simulink model "SPM_Pack"  (R2024b)
settings: Solver=VariableStepAuto  StartTime=0.0  StopTime=10.0  RelTol=1e-3
libraries: fl_lib x74, nesl_utility x33, batt_lib x8, BatteryEstimators x8, ee_lib x8
(part 1 of 2)
settings Model: Creator=annaf  LastModifiedBy=annaf

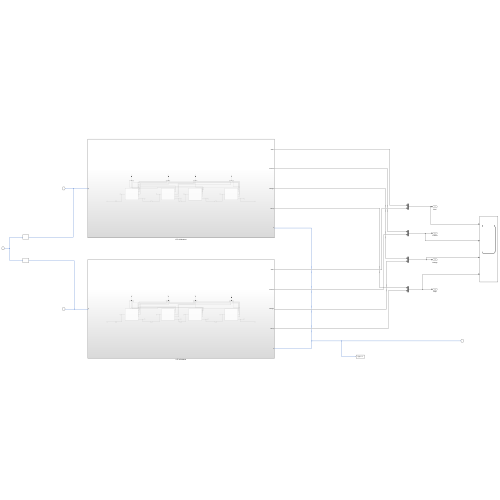
[thumbnail: Simulink's stored preview of the top-level diagram]
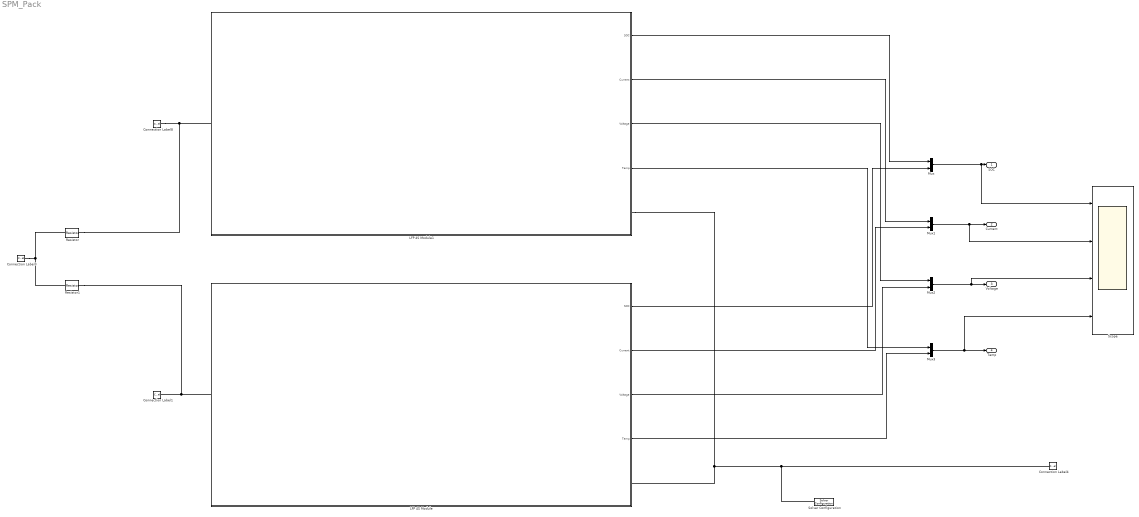
== system SPM_Pack ==
  Connection Label1 : ConnectionLabel  Label=p
  Connection Label3 : ConnectionLabel  Label=p
  Connection Label4 : ConnectionLabel  Label=n
  Connection Label8 : ConnectionLabel  Label=p
  LFP 4S Module : Subsystem
  LFP 4S Module1 : Subsystem
  Mux{,1..3} (4 alike) : Mux  Inputs=2
  Resistor : fl_lib/Electrical/Electrical Elements/Resistor  R=0.001 Ohm  i_specify=off  i_priority=None  i=0 A  i_nominal_specify=off  i_nominal_value=1  i_nominal_unit=A  v_specify=off  v_priority=None  v=0 V  v_nominal_specify=off  v_nominal_value=1  v_nominal_unit=V
  Resistor1 : fl_lib/Electrical/Electrical Elements/Resistor  R=0.001 Ohm  i_specify=off  i_priority=None  i=0 A  i_nominal_specify=off  i_nominal_value=1  i_nominal_unit=A  v_specify=off  v_priority=None  v=0 V  v_nominal_specify=off  v_nominal_value=1  v_nominal_unit=V
  Scope : Scope  NumInputPorts=4
  Solver Configuration : nesl_utility/Solver Configuration  PhysicalDomain=network_engine_domain  SubClassName=solver  LeftPortType=input  RightPortType=generic  Tones=[]  Harmonics=[]  SimulateNoise=off  Profile=off  UseLocalSampling=off  EnableSwitchedLinearOptims=on  FrequencyDomain=off  UseCCode=off  RelTol=0.001  AbsTol=0.001  MinStep=1e-09  ToWorkspace=off  RevertToSquareIcSolve=off  NumHomotopyIterations=100  PhasorMode=off  PhasorModeNumHarmonics=1  ConsistencySolver=NEWTON_XTOL_AFTER_FTOL  IndexReductionMethod=DerivativeReplacement  DoDC=off  ResidualTolerance=1e-09  ConsistencyTolSource=GLOBAL  ConsistencyAbsTol=0.001  ConsistencyRelTol=0.001  ConsistencyTolFactor=0.001  UseLocalSolver=on  LocalSolverChoice=NE_BACKWARD_EULER_ADVANCER  ResolveIndetEquations=off  FunctionEvalNumThread=1  LocalSolverSampleTime=0.1  DoFixedCost=off  MaxNonlinIter=3  MaxModeIter=2  ComputeImpulses=off  ImpulseIterations=2  LinearAlgebra=auto  LinearAlgebraNumThread=0  EquationFormulation=NE_TIME_EF  DelaysMemoryBudget=1024  AutomaticFiltering=on  FilteringTimeConstant=0.001  PartitionStorageMethod=AS_NEEDED  PartitionMemoryBudget=1024  PartitionMethod=ROBUST  MultibodyUseLocalSolver=off  MultibodyLocalSolverChoice=ODE1  MultibodyLocalSolverSampleTime=0.001
  SOC : Outport
  Current : Outport  Port=2
  Voltage : Outport  Port=3
  Temp : Outport  Port=4
  wires:
  Mux2/1 -> Scope/3, Voltage/1
  Mux1/1 -> Scope/2, Current/1
  Mux/1 -> Scope/1, SOC/1
  Mux3/1 -> Scope/4, Temp/1
  LFP 4S Module1/1(SOC) -> Mux/1
  LFP 4S Module/1(SOC) -> Mux/2
  LFP 4S Module1/2(Current) -> Mux1/1
  LFP 4S Module1/3(Voltage) -> Mux2/1
  LFP 4S Module1/4(Temp) -> Mux3/1
  LFP 4S Module/2(Current) -> Mux1/2
  LFP 4S Module/3(Voltage) -> Mux2/2
  LFP 4S Module/4(Temp) -> Mux3/2
  connections:
  Connection Label8/LConn1 -- Resistor/RConn1 -- LFP 4S Module1/LConn1
  LFP 4S Module1/RConn1 -- Solver Configuration/RConn1 -- Connection Label4/LConn1 -- LFP 4S Module/RConn1
  LFP 4S Module/LConn1 -- Resistor1/RConn1 -- Connection Label1/LConn1
  Resistor1/LConn1 -- Connection Label3/LConn1 -- Resistor/LConn1

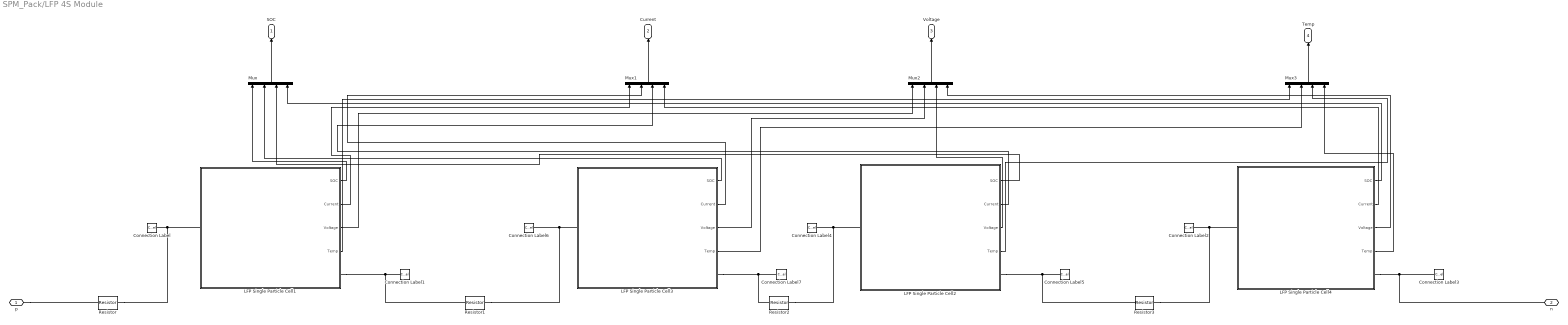
== system SPM_Pack/LFP 4S Module ==
  Connection Label{,2,4,6} (4 alike) : ConnectionLabel  Label=p
  Connection Label{1,3,5,7} (4 alike) : ConnectionLabel  Label=n
  LFP Single Particle Cell1 : Subsystem
  LFP Single Particle Cell2 : Subsystem
  LFP Single Particle Cell3 : Subsystem
  LFP Single Particle Cell4 : Subsystem
  Mux{,1..3} (4 alike) : Mux
  Resistor : ee_lib/Passive/Resistor  R=0.002 Ohm  enable_R_tol=ee.enum.toleranceApplication.none  R_tol=5  tol_distribution=ee.enum.toleranceDistribution.uniform  nSigma=4  enable_operating_limits=ee.enum.enable.no  operating_limit_action=ee.enum.passive.reportOpLim.warn  power_rating=1 W  max_working_voltage=100 V  noise_mode=ee.enum.sources.noise.Disabled  Tdevice=25 degC  sample_time=1e-3 s  repeatability=ee.enum.ic.repeatability.notRepeatable  user_seed=0  auto_seed=4144164703  fault_action=simscape.enum.assert.action.none  t_fault=1 s  power_derating_T1=70 degC  power_derating_T2=155 degC  operating_temperature_range_vec=[-50, 150] degC  alpha=3.93e-3 1/K  Tmeas=25 degC  thermal_mass=100 J/K  temperature_specify=off  temperature_priority=High  temperature=298.15 K  temperature_nominal_specify=off  temperature_nominal_value=1  temperature_nominal_unit=K
  Resistor1 : ee_lib/Passive/Resistor  R=0.002 Ohm  enable_R_tol=ee.enum.toleranceApplication.none  R_tol=5  tol_distribution=ee.enum.toleranceDistribution.uniform  nSigma=4  enable_operating_limits=ee.enum.enable.no  operating_limit_action=ee.enum.passive.reportOpLim.warn  power_rating=1 W  max_working_voltage=100 V  noise_mode=ee.enum.sources.noise.Disabled  Tdevice=25 degC  sample_time=1e-3 s  repeatability=ee.enum.ic.repeatability.notRepeatable  user_seed=0  auto_seed=676943032  fault_action=simscape.enum.assert.action.none  t_fault=1 s  power_derating_T1=70 degC  power_derating_T2=155 degC  operating_temperature_range_vec=[-50, 150] degC  alpha=3.93e-3 1/K  Tmeas=25 degC  thermal_mass=100 J/K  temperature_specify=off  temperature_priority=High  temperature=298.15 K  temperature_nominal_specify=off  temperature_nominal_value=1  temperature_nominal_unit=K
  Resistor2 : ee_lib/Passive/Resistor  R=0.002 Ohm  enable_R_tol=ee.enum.toleranceApplication.none  R_tol=5  tol_distribution=ee.enum.toleranceDistribution.uniform  nSigma=4  enable_operating_limits=ee.enum.enable.no  operating_limit_action=ee.enum.passive.reportOpLim.warn  power_rating=1 W  max_working_voltage=100 V  noise_mode=ee.enum.sources.noise.Disabled  Tdevice=25 degC  sample_time=1e-3 s  repeatability=ee.enum.ic.repeatability.notRepeatable  user_seed=0  auto_seed=4168664255  fault_action=simscape.enum.assert.action.none  t_fault=1 s  power_derating_T1=70 degC  power_derating_T2=155 degC  operating_temperature_range_vec=[-50, 150] degC  alpha=3.93e-3 1/K  Tmeas=25 degC  thermal_mass=100 J/K  temperature_specify=off  temperature_priority=High  temperature=298.15 K  temperature_nominal_specify=off  temperature_nominal_value=1  temperature_nominal_unit=K
  Resistor3 : ee_lib/Passive/Resistor  R=0.002 Ohm  enable_R_tol=ee.enum.toleranceApplication.none  R_tol=5  tol_distribution=ee.enum.toleranceDistribution.uniform  nSigma=4  enable_operating_limits=ee.enum.enable.no  operating_limit_action=ee.enum.passive.reportOpLim.warn  power_rating=1 W  max_working_voltage=100 V  noise_mode=ee.enum.sources.noise.Disabled  Tdevice=25 degC  sample_time=1e-3 s  repeatability=ee.enum.ic.repeatability.notRepeatable  user_seed=0  auto_seed=4111000739  fault_action=simscape.enum.assert.action.none  t_fault=1 s  power_derating_T1=70 degC  power_derating_T2=155 degC  operating_temperature_range_vec=[-50, 150] degC  alpha=3.93e-3 1/K  Tmeas=25 degC  thermal_mass=100 J/K  temperature_specify=off  temperature_priority=High  temperature=298.15 K  temperature_nominal_specify=off  temperature_nominal_value=1  temperature_nominal_unit=K
  p : PMIOPort  Side=Left
  n : PMIOPort  Port=2  Side=Right
  SOC : Outport
  Current : Outport  Port=2
  Voltage : Outport  Port=3
  Temp : Outport  Port=4
  wires:
  LFP Single Particle Cell1/1(SOC) -> Mux/1
  LFP Single Particle Cell4/4(Temp) -> Mux3/4
  LFP Single Particle Cell2/3(Voltage) -> Mux2/3
  LFP Single Particle Cell3/2(Current) -> Mux1/2
  LFP Single Particle Cell1/2(Current) -> Mux1/1
  LFP Single Particle Cell1/3(Voltage) -> Mux2/1
  LFP Single Particle Cell4/3(Voltage) -> Mux2/4
  LFP Single Particle Cell2/4(Temp) -> Mux3/3
  Mux3/1 -> Temp/1
  LFP Single Particle Cell4/1(SOC) -> Mux/4
  LFP Single Particle Cell2/1(SOC) -> Mux/3
  LFP Single Particle Cell3/3(Voltage) -> Mux2/2
  Mux/1 -> SOC/1
  LFP Single Particle Cell2/2(Current) -> Mux1/3
  LFP Single Particle Cell4/2(Current) -> Mux1/4
  LFP Single Particle Cell3/4(Temp) -> Mux3/2
  Mux2/1 -> Voltage/1
  Mux1/1 -> Current/1
  LFP Single Particle Cell3/1(SOC) -> Mux/2
  LFP Single Particle Cell1/4(Temp) -> Mux3/1
  connections:
  LFP Single Particle Cell4/RConn1 -- Connection Label3/LConn1 -- n/RConn1
  LFP Single Particle Cell3/RConn1 -- Connection Label7/LConn1 -- Resistor2/LConn1
  LFP Single Particle Cell2/LConn1 -- Connection Label4/LConn1 -- Resistor2/RConn1
  LFP Single Particle Cell1/LConn1 -- Connection Label/LConn1 -- Resistor/RConn1
  LFP Single Particle Cell4/LConn1 -- Connection Label2/LConn1 -- Resistor3/RConn1
  LFP Single Particle Cell1/RConn1 -- Connection Label1/LConn1 -- Resistor1/LConn1
  LFP Single Particle Cell3/LConn1 -- Connection Label6/LConn1 -- Resistor1/RConn1
  LFP Single Particle Cell2/RConn1 -- Connection Label5/LConn1 -- Resistor3/LConn1
  p/RConn1 -- Resistor/LConn1

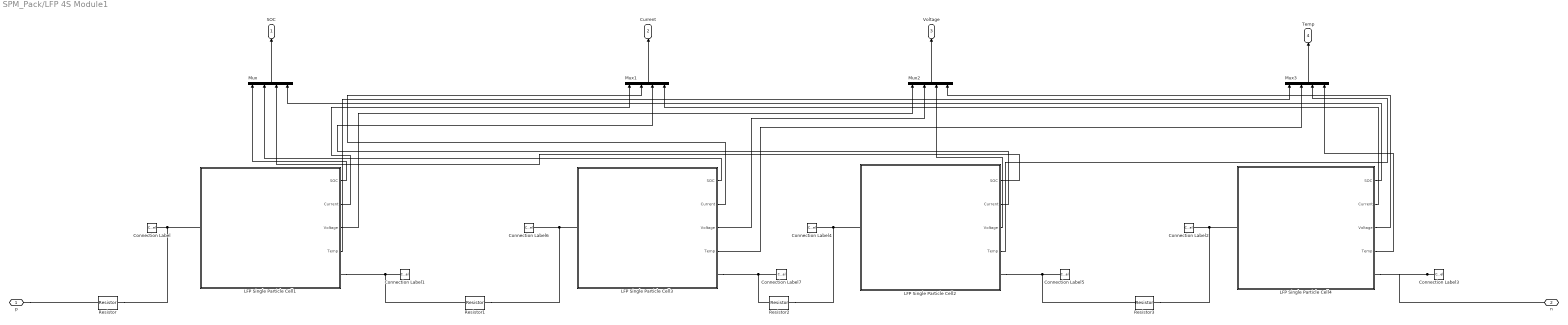
== system SPM_Pack/LFP 4S Module1 ==
  Connection Label{,2,4,6} (4 alike) : ConnectionLabel  Label=p
  Connection Label{1,3,5,7} (4 alike) : ConnectionLabel  Label=n
  LFP Single Particle Cell1 : Subsystem
  LFP Single Particle Cell2 : Subsystem
  LFP Single Particle Cell3 : Subsystem
  LFP Single Particle Cell4 : Subsystem
  Mux{,1..3} (4 alike) : Mux
  Resistor : ee_lib/Passive/Resistor  R=0.002 Ohm  enable_R_tol=ee.enum.toleranceApplication.none  R_tol=5  tol_distribution=ee.enum.toleranceDistribution.uniform  nSigma=4  enable_operating_limits=ee.enum.enable.no  operating_limit_action=ee.enum.passive.reportOpLim.warn  power_rating=1 W  max_working_voltage=100 V  noise_mode=ee.enum.sources.noise.Disabled  Tdevice=25 degC  sample_time=1e-3 s  repeatability=ee.enum.ic.repeatability.notRepeatable  user_seed=0  auto_seed=418932850  fault_action=simscape.enum.assert.action.none  t_fault=1 s  power_derating_T1=70 degC  power_derating_T2=155 degC  operating_temperature_range_vec=[-50, 150] degC  alpha=3.93e-3 1/K  Tmeas=25 degC  thermal_mass=100 J/K  temperature_specify=off  temperature_priority=High  temperature=298.15 K  temperature_nominal_specify=off  temperature_nominal_value=1  temperature_nominal_unit=K
  Resistor1 : ee_lib/Passive/Resistor  R=0.002 Ohm  enable_R_tol=ee.enum.toleranceApplication.none  R_tol=5  tol_distribution=ee.enum.toleranceDistribution.uniform  nSigma=4  enable_operating_limits=ee.enum.enable.no  operating_limit_action=ee.enum.passive.reportOpLim.warn  power_rating=1 W  max_working_voltage=100 V  noise_mode=ee.enum.sources.noise.Disabled  Tdevice=25 degC  sample_time=1e-3 s  repeatability=ee.enum.ic.repeatability.notRepeatable  user_seed=0  auto_seed=1196140742  fault_action=simscape.enum.assert.action.none  t_fault=1 s  power_derating_T1=70 degC  power_derating_T2=155 degC  operating_temperature_range_vec=[-50, 150] degC  alpha=3.93e-3 1/K  Tmeas=25 degC  thermal_mass=100 J/K  temperature_specify=off  temperature_priority=High  temperature=298.15 K  temperature_nominal_specify=off  temperature_nominal_value=1  temperature_nominal_unit=K
  Resistor2 : ee_lib/Passive/Resistor  R=0.002 Ohm  enable_R_tol=ee.enum.toleranceApplication.none  R_tol=5  tol_distribution=ee.enum.toleranceDistribution.uniform  nSigma=4  enable_operating_limits=ee.enum.enable.no  operating_limit_action=ee.enum.passive.reportOpLim.warn  power_rating=1 W  max_working_voltage=100 V  noise_mode=ee.enum.sources.noise.Disabled  Tdevice=25 degC  sample_time=1e-3 s  repeatability=ee.enum.ic.repeatability.notRepeatable  user_seed=0  auto_seed=2348838240  fault_action=simscape.enum.assert.action.none  t_fault=1 s  power_derating_T1=70 degC  power_derating_T2=155 degC  operating_temperature_range_vec=[-50, 150] degC  alpha=3.93e-3 1/K  Tmeas=25 degC  thermal_mass=100 J/K  temperature_specify=off  temperature_priority=High  temperature=298.15 K  temperature_nominal_specify=off  temperature_nominal_value=1  temperature_nominal_unit=K
  Resistor3 : ee_lib/Passive/Resistor  R=0.002 Ohm  enable_R_tol=ee.enum.toleranceApplication.none  R_tol=5  tol_distribution=ee.enum.toleranceDistribution.uniform  nSigma=4  enable_operating_limits=ee.enum.enable.no  operating_limit_action=ee.enum.passive.reportOpLim.warn  power_rating=1 W  max_working_voltage=100 V  noise_mode=ee.enum.sources.noise.Disabled  Tdevice=25 degC  sample_time=1e-3 s  repeatability=ee.enum.ic.repeatability.notRepeatable  user_seed=0  auto_seed=4112460543  fault_action=simscape.enum.assert.action.none  t_fault=1 s  power_derating_T1=70 degC  power_derating_T2=155 degC  operating_temperature_range_vec=[-50, 150] degC  alpha=3.93e-3 1/K  Tmeas=25 degC  thermal_mass=100 J/K  temperature_specify=off  temperature_priority=High  temperature=298.15 K  temperature_nominal_specify=off  temperature_nominal_value=1  temperature_nominal_unit=K
  p : PMIOPort  Side=Left
  n : PMIOPort  Port=2  Side=Right
  SOC : Outport
  Current : Outport  Port=2
  Voltage : Outport  Port=3
  Temp : Outport  Port=4
  wires:
  LFP Single Particle Cell1/1(SOC) -> Mux/1
  LFP Single Particle Cell4/4(Temp) -> Mux3/4
  LFP Single Particle Cell2/3(Voltage) -> Mux2/3
  LFP Single Particle Cell3/2(Current) -> Mux1/2
  LFP Single Particle Cell1/2(Current) -> Mux1/1
  LFP Single Particle Cell1/3(Voltage) -> Mux2/1
  LFP Single Particle Cell4/3(Voltage) -> Mux2/4
  LFP Single Particle Cell2/4(Temp) -> Mux3/3
  Mux3/1 -> Temp/1
  LFP Single Particle Cell4/1(SOC) -> Mux/4
  LFP Single Particle Cell2/1(SOC) -> Mux/3
  LFP Single Particle Cell3/3(Voltage) -> Mux2/2
  Mux/1 -> SOC/1
  LFP Single Particle Cell2/2(Current) -> Mux1/3
  LFP Single Particle Cell4/2(Current) -> Mux1/4
  LFP Single Particle Cell3/4(Temp) -> Mux3/2
  Mux2/1 -> Voltage/1
  Mux1/1 -> Current/1
  LFP Single Particle Cell3/1(SOC) -> Mux/2
  LFP Single Particle Cell1/4(Temp) -> Mux3/1
  connections:
  Connection Label3/LConn1 -- n/RConn1 -- LFP Single Particle Cell4/RConn1
  LFP Single Particle Cell3/RConn1 -- Resistor2/LConn1 -- Connection Label7/LConn1
  LFP Single Particle Cell2/LConn1 -- Resistor2/RConn1 -- Connection Label4/LConn1
  LFP Single Particle Cell1/LConn1 -- Resistor/RConn1 -- Connection Label/LConn1
  LFP Single Particle Cell4/LConn1 -- Resistor3/RConn1 -- Connection Label2/LConn1
  LFP Single Particle Cell1/RConn1 -- Resistor1/LConn1 -- Connection Label1/LConn1
  LFP Single Particle Cell3/LConn1 -- Resistor1/RConn1 -- Connection Label6/LConn1
  LFP Single Particle Cell2/RConn1 -- Resistor3/LConn1 -- Connection Label5/LConn1
  p/RConn1 -- Resistor/LConn1

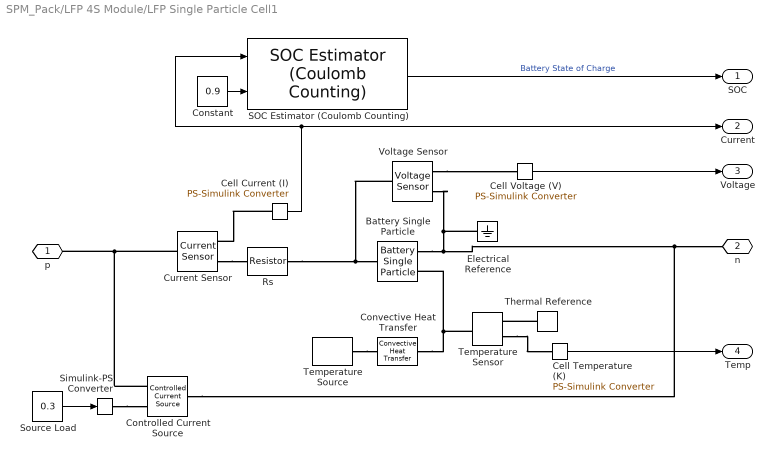
== system SPM_Pack/LFP 4S Module/LFP Single Particle Cell1 ==
  Battery Single Particle : batt_lib/Cells/Electrochemical/Battery Single Particle  ExtrapolationMethod=simscape.enum.extrapolation.nearest  ThicknessAnode=3.4E-5 m  ElectrolyteLayerCountAnode=10  ThicknessSeparator=2.5E-5 m  ElectrolyteLayerCountSeparator=5  ThicknessCathode=8E-5 m  ElectrolyteLayerCountCathode=10  ElectrodePlateArea=0.2 m^2  ParticleRadiusAnode=5E-6 m  ShellCountAnode=30  ParticleRadiusCathode=5E-6 m  ShellCountCathode=30  ActiveMaterialVolumeFractionAnode=0.58  ActiveMaterialVolumeFractionCathode=0.374  OpenCircuitPotentialAnode=[0.200;0.180;0.160;0.140;0.120;0.110;0.102;0.098;0.094;0.092;0.091;0.090;0.089;0.089;0.088;0.088;0.088;0.088;0.088;0.088;0.088;0.087;0.087;0.087;0.086;0.086;0.085;0.085;0.084;0.084;0.083;0.083;0.082;0.082;0.081;0.081;0.080;0.079;0.078] V  OpenCircuitPotentialCathode=[3.200;3.280;3.340;3.380;3.410;3.420;3.425;3.430;3.432;3.433;3.434;3.435;3.435;3.436;3.436;3.437;3.437;3.438;3.438;3.439;3.439;3.440;3.440;3.441;3.441;3.442;3.442;3.443;3.443;3.444;3.444;3.445;3.446;3.447;3.448;3.449;3.460;3.480;3.500] V  NormalizedStoichiometryBreakpoints=linspace(0.025, 0.975, 39)  MaximumConcentrationAnode=30555 mol/m^3  MaximumStoichiometryAnode=0.811  MinimumStoichiometryAnode=0.0132  MaximumConcentrationCathode=22806 mol/m^3  MaximumStoichiometryCathode=0.74  MinimumStoichiometryCathode=0.035  ActiveMaterialDiffusionCoefficientAnode=3E-15 m^2/s  ActiveMaterialDiffusionCoefficientCathode=1E-15 m^2/s  ConductivityAnode=100 S/m  ConductivityCathode=0.5 S/m  CurrentCollectorResistance=1E-3 Ohm  ElectrolyteVolumeFractionAnode=0.3874  ElectrolyteVolumeFractionSeparator=0.45  ElectrolyteVolumeFractionCathode=0.5725  ElectrolyteConductivity=0.29 S/m  BruggemanExponentAnode=1.5  BruggemanExponentSeparator=1.5  BruggemanExponentCathode=1.5  TransferenceNumber=0.363  ElectrolyteDiffusionCoefficient=2E-10 m^2/s  ChargeTransferRateAnode=1E-9 m^(5/2)/(mol^(1/2)*s)  ChargeTransferRateCathode=1E-11 m^(5/2)/(mol^(1/2)*s)  BatteryThermalMass=77 J/K  ArrheniusReferenceTemperature=298.15 K  ActiveMaterialDiffusionActivationEnergyAnode=39000 J/mol  ActiveMaterialDiffusionActivationEnergyCathode=35000 J/mol  ElectrolyteDiffusionActivationEnergy=26600 J/mol  ConductivityActivationEnergyAnode=3000 J/mol  ConductivityActivationEnergyCathode=3000 J/mol  ElectrolyteConductivityActivationEnergy=11000 J/mol  ChargeTransferActivationEnergyAnode=13000 J/mol  ChargeTransferActivationEnergyCathode=20000 J/mol  batteryCurrent_specify=off  batteryCurrent_priority=None  batteryCurrent=0 A  batteryCurrent_nominal_specify=off  batteryCurrent_nominal_value=1  batteryCurrent_nominal_unit=A  batteryVoltage_specify=off  batteryVoltage_priority=None  batteryVoltage=0 V  batteryVoltage_nominal_specify=off  batteryVoltage_nominal_value=1  batteryVoltage_nominal_unit=V  averageElectrolyteConcentration_specify=off  averageElectrolyteConcentration_priority=High  averageElectrolyteConcentration=1200 mol/m^3  averageElectrolyteConcentration_nominal_specify=off  averageElectrolyteConcentration_nominal_value=1  averageElectrolyteConcentration_nominal_unit=mol/m^3  stateOfCharge_specify=off  stateOfCharge_priority=High  stateOfCharge=0.5  stateOfCharge_nominal_specify=off  stateOfCharge_nominal_value=1  stateOfCharge_nominal_unit=1  batteryTemperature_specify=off  batteryTemperature_priority=High  batteryTemperature=298.15 K  batteryTemperature_nominal_specify=off  batteryTemperature_nominal_value=1  batteryTemperature_nominal_unit=K
      settings: InternalSimscapePortConfiguration="{\"Bottom\":[],\"Left\":[{\"id\":\"p\",\"label\":\"+\",\"type\":\"foundation.electrical.electrical\"}],\"Right\":[{\"id\":\"n\",\"label\":\"-\",\"type\":\"foundation.electrical.electrical\"},{\"id\":\"H\",\"label\":\"H\",\"type\":\"foundation.thermal.thermal\"}],\"Top\":[]}"
  Cell Current (I) : nesl_utility/PS-Simulink Converter  PhysicalDomain=network_engine_domain  SubClassName=ps_output  LeftPortType=input  RightPortType=output  PseudoPeriodic=off  Frequencies=[]  VectorFormat=inherit  Unit=A  AffineConversion=off
  Cell Temperature (K) : nesl_utility/PS-Simulink Converter  PhysicalDomain=network_engine_domain  SubClassName=ps_output  LeftPortType=input  RightPortType=output  PseudoPeriodic=off  Frequencies=[]  VectorFormat=inherit  Unit=K  AffineConversion=off
  Cell Voltage (V) : nesl_utility/PS-Simulink Converter  PhysicalDomain=network_engine_domain  SubClassName=ps_output  LeftPortType=input  RightPortType=output  PseudoPeriodic=off  Frequencies=[]  VectorFormat=inherit  Unit=V  AffineConversion=off
  Constant : Constant  Value=0.9
  Controlled Current Source : fl_lib/Electrical/Electrical Sources/Controlled Current Source
  Convective Heat Transfer : fl_lib/Thermal/Thermal Elements/Convective Heat Transfer  thermal_type=foundation.enum.constant_variable.constant  area=0.01 m^2  heat_tr_coeff=15 W/(K*m^2)  min_heat_tr_coeff=1e-3 W/(K*m^2)  T_specify=off  T_priority=None  T=0 K  T_nominal_specify=off  T_nominal_value=1  T_nominal_unit=K  Q_specify=off  Q_priority=None  Q=0 W  Q_nominal_specify=off  Q_nominal_value=1  Q_nominal_unit=W
  Current Sensor : fl_lib/Electrical/Electrical Sensors/Current Sensor
  Electrical Reference : fl_lib/Electrical/Electrical Elements/Electrical Reference
  Rs : fl_lib/Electrical/Electrical Elements/Resistor  R=0.004 Ohm  i_specify=off  i_priority=None  i=0 A  i_nominal_specify=off  i_nominal_value=3  i_nominal_unit=A  v_specify=off  v_priority=None  v=0 V  v_nominal_specify=off  v_nominal_value=3.5  v_nominal_unit=V
  SOC Estimator (Coulomb Counting) : BatteryEstimators/SOC Estimator (Coulomb Counting)  CurrentInputPartition=on  AH=27  Ts=1
      settings: LibrarySourceBlock=|
      | batt_sl_lib/Estimators/SOC Estimator
      | (Coulomb Counting)
  Simulink-PS Converter : nesl_utility/Simulink-PS Converter  PhysicalDomain=network_engine_domain  SubClassName=ps_input  LeftPortType=input  RightPortType=output  PseudoPeriodic=off  Frequencies=[]  NoiseDistribution=none  NoiseParameters=[]  Unit=A  AffineConversion=off  FilteringAndDerivatives=provide  SimscapeFilterOrder=1  InputFilterTimeConstant=0.001  UdotUserProvided=0
  Source Load : Constant  Value=0.3
  Temperature Sensor : fl_lib/Thermal/Thermal Sensors/Temperature Sensor  temperature_measure=foundation.enum.MeasurementReference.difference
  Temperature Source : fl_lib/Thermal/Thermal Sources/Temperature Source  temperature=298.15 K
  Thermal Reference : fl_lib/Thermal/Thermal Elements/Thermal Reference
  Voltage Sensor : fl_lib/Electrical/Electrical Sensors/Voltage Sensor
  p : PMIOPort  Side=Left
  n : PMIOPort  Port=2  Side=Right
  SOC : Outport
  Current : Outport  Port=2
  Voltage : Outport  Port=3
  Temp : Outport  Port=4
  wires:
  Cell Current (I)/1 -> Current/1, SOC Estimator (Coulomb Counting)/1
  SOC Estimator (Coulomb Counting)/1 -> SOC/1  "Battery State of Charge"
  Constant/1 -> SOC Estimator (Coulomb Counting)/2
  Cell Voltage (V)/1 -> Voltage/1
  Cell Temperature (K)/1 -> Temp/1
  Source Load/1 -> Simulink-PS Converter/1
  connections:
  Temperature Sensor/RConn2 -- Cell Temperature (K)/LConn1
  Voltage Sensor/RConn1 -- Cell Voltage (V)/LConn1
  Temperature Sensor/LConn1 -- Battery Single Particle/RConn2 -- Convective Heat Transfer/LConn1
  Thermal Reference/LConn1 -- Temperature Sensor/RConn1
  Temperature Source/LConn1 -- Convective Heat Transfer/RConn1
  Rs/LConn1 -- Voltage Sensor/LConn1 -- Battery Single Particle/LConn1
  Battery Single Particle/RConn1 -- Voltage Sensor/RConn2 -- Electrical Reference/LConn1 -- Controlled Current Source/LConn1 -- n/RConn1
  Cell Current (I)/LConn1 -- Current Sensor/RConn1
  Current Sensor/LConn1 -- Controlled Current Source/RConn2 -- p/RConn1
  Simulink-PS Converter/RConn1 -- Controlled Current Source/RConn1
  Current Sensor/RConn2 -- Rs/RConn1

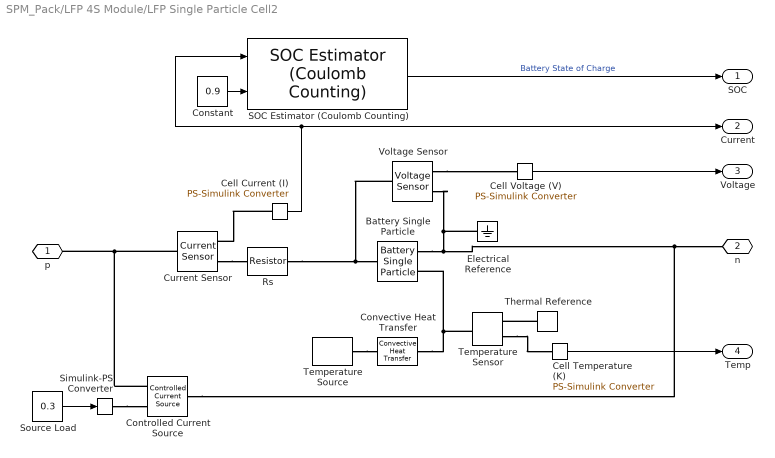
== system SPM_Pack/LFP 4S Module/LFP Single Particle Cell2 ==
  Battery Single Particle : batt_lib/Cells/Electrochemical/Battery Single Particle  ExtrapolationMethod=simscape.enum.extrapolation.nearest  ThicknessAnode=3.4E-5 m  ElectrolyteLayerCountAnode=10  ThicknessSeparator=2.5E-5 m  ElectrolyteLayerCountSeparator=5  ThicknessCathode=8E-5 m  ElectrolyteLayerCountCathode=10  ElectrodePlateArea=0.2 m^2  ParticleRadiusAnode=5E-6 m  ShellCountAnode=30  ParticleRadiusCathode=5E-6 m  ShellCountCathode=30  ActiveMaterialVolumeFractionAnode=0.58  ActiveMaterialVolumeFractionCathode=0.374  OpenCircuitPotentialAnode=[0.200;0.180;0.160;0.140;0.120;0.110;0.102;0.098;0.094;0.092;0.091;0.090;0.089;0.089;0.088;0.088;0.088;0.088;0.088;0.088;0.088;0.087;0.087;0.087;0.086;0.086;0.085;0.085;0.084;0.084;0.083;0.083;0.082;0.082;0.081;0.081;0.080;0.079;0.078] V  OpenCircuitPotentialCathode=[3.200;3.280;3.340;3.380;3.410;3.420;3.425;3.430;3.432;3.433;3.434;3.435;3.435;3.436;3.436;3.437;3.437;3.438;3.438;3.439;3.439;3.440;3.440;3.441;3.441;3.442;3.442;3.443;3.443;3.444;3.444;3.445;3.446;3.447;3.448;3.449;3.460;3.480;3.500] V  NormalizedStoichiometryBreakpoints=linspace(0.025, 0.975, 39)  MaximumConcentrationAnode=30555 mol/m^3  MaximumStoichiometryAnode=0.811  MinimumStoichiometryAnode=0.0132  MaximumConcentrationCathode=22806 mol/m^3  MaximumStoichiometryCathode=0.74  MinimumStoichiometryCathode=0.035  ActiveMaterialDiffusionCoefficientAnode=3E-15 m^2/s  ActiveMaterialDiffusionCoefficientCathode=1E-15 m^2/s  ConductivityAnode=100 S/m  ConductivityCathode=0.5 S/m  CurrentCollectorResistance=1E-3 Ohm  ElectrolyteVolumeFractionAnode=0.3874  ElectrolyteVolumeFractionSeparator=0.45  ElectrolyteVolumeFractionCathode=0.5725  ElectrolyteConductivity=0.29 S/m  BruggemanExponentAnode=1.5  BruggemanExponentSeparator=1.5  BruggemanExponentCathode=1.5  TransferenceNumber=0.363  ElectrolyteDiffusionCoefficient=2E-10 m^2/s  ChargeTransferRateAnode=1E-9 m^(5/2)/(mol^(1/2)*s)  ChargeTransferRateCathode=1E-11 m^(5/2)/(mol^(1/2)*s)  BatteryThermalMass=77 J/K  ArrheniusReferenceTemperature=298.15 K  ActiveMaterialDiffusionActivationEnergyAnode=39000 J/mol  ActiveMaterialDiffusionActivationEnergyCathode=35000 J/mol  ElectrolyteDiffusionActivationEnergy=26600 J/mol  ConductivityActivationEnergyAnode=3000 J/mol  ConductivityActivationEnergyCathode=3000 J/mol  ElectrolyteConductivityActivationEnergy=11000 J/mol  ChargeTransferActivationEnergyAnode=13000 J/mol  ChargeTransferActivationEnergyCathode=20000 J/mol  batteryCurrent_specify=off  batteryCurrent_priority=None  batteryCurrent=0 A  batteryCurrent_nominal_specify=off  batteryCurrent_nominal_value=1  batteryCurrent_nominal_unit=A  batteryVoltage_specify=off  batteryVoltage_priority=None  batteryVoltage=0 V  batteryVoltage_nominal_specify=off  batteryVoltage_nominal_value=1  batteryVoltage_nominal_unit=V  averageElectrolyteConcentration_specify=off  averageElectrolyteConcentration_priority=High  averageElectrolyteConcentration=1200 mol/m^3  averageElectrolyteConcentration_nominal_specify=off  averageElectrolyteConcentration_nominal_value=1  averageElectrolyteConcentration_nominal_unit=mol/m^3  stateOfCharge_specify=off  stateOfCharge_priority=High  stateOfCharge=0.5  stateOfCharge_nominal_specify=off  stateOfCharge_nominal_value=1  stateOfCharge_nominal_unit=1  batteryTemperature_specify=off  batteryTemperature_priority=High  batteryTemperature=298.15 K  batteryTemperature_nominal_specify=off  batteryTemperature_nominal_value=1  batteryTemperature_nominal_unit=K
      settings: InternalSimscapePortConfiguration="{\"Bottom\":[],\"Left\":[{\"id\":\"p\",\"label\":\"+\",\"type\":\"foundation.electrical.electrical\"}],\"Right\":[{\"id\":\"n\",\"label\":\"-\",\"type\":\"foundation.electrical.electrical\"},{\"id\":\"H\",\"label\":\"H\",\"type\":\"foundation.thermal.thermal\"}],\"Top\":[]}"
  Cell Current (I) : nesl_utility/PS-Simulink Converter  PhysicalDomain=network_engine_domain  SubClassName=ps_output  LeftPortType=input  RightPortType=output  PseudoPeriodic=off  Frequencies=[]  VectorFormat=inherit  Unit=A  AffineConversion=off
  Cell Temperature (K) : nesl_utility/PS-Simulink Converter  PhysicalDomain=network_engine_domain  SubClassName=ps_output  LeftPortType=input  RightPortType=output  PseudoPeriodic=off  Frequencies=[]  VectorFormat=inherit  Unit=K  AffineConversion=off
  Cell Voltage (V) : nesl_utility/PS-Simulink Converter  PhysicalDomain=network_engine_domain  SubClassName=ps_output  LeftPortType=input  RightPortType=output  PseudoPeriodic=off  Frequencies=[]  VectorFormat=inherit  Unit=V  AffineConversion=off
  Constant : Constant  Value=0.9
  Controlled Current Source : fl_lib/Electrical/Electrical Sources/Controlled Current Source
  Convective Heat Transfer : fl_lib/Thermal/Thermal Elements/Convective Heat Transfer  thermal_type=foundation.enum.constant_variable.constant  area=0.01 m^2  heat_tr_coeff=15 W/(K*m^2)  min_heat_tr_coeff=1e-3 W/(K*m^2)  T_specify=off  T_priority=None  T=0 K  T_nominal_specify=off  T_nominal_value=1  T_nominal_unit=K  Q_specify=off  Q_priority=None  Q=0 W  Q_nominal_specify=off  Q_nominal_value=1  Q_nominal_unit=W
  Current Sensor : fl_lib/Electrical/Electrical Sensors/Current Sensor
  Electrical Reference : fl_lib/Electrical/Electrical Elements/Electrical Reference
  Rs : fl_lib/Electrical/Electrical Elements/Resistor  R=0.004 Ohm  i_specify=off  i_priority=None  i=0 A  i_nominal_specify=off  i_nominal_value=3  i_nominal_unit=A  v_specify=off  v_priority=None  v=0 V  v_nominal_specify=off  v_nominal_value=3.5  v_nominal_unit=V
  SOC Estimator (Coulomb Counting) : BatteryEstimators/SOC Estimator (Coulomb Counting)  CurrentInputPartition=on  AH=27  Ts=1
      settings: LibrarySourceBlock=|
      | batt_sl_lib/Estimators/SOC Estimator
      | (Coulomb Counting)
  Simulink-PS Converter : nesl_utility/Simulink-PS Converter  PhysicalDomain=network_engine_domain  SubClassName=ps_input  LeftPortType=input  RightPortType=output  PseudoPeriodic=off  Frequencies=[]  NoiseDistribution=none  NoiseParameters=[]  Unit=A  AffineConversion=off  FilteringAndDerivatives=provide  SimscapeFilterOrder=1  InputFilterTimeConstant=0.001  UdotUserProvided=0
  Source Load : Constant  Value=0.3
  Temperature Sensor : fl_lib/Thermal/Thermal Sensors/Temperature Sensor  temperature_measure=foundation.enum.MeasurementReference.difference
  Temperature Source : fl_lib/Thermal/Thermal Sources/Temperature Source  temperature=298.15 K
  Thermal Reference : fl_lib/Thermal/Thermal Elements/Thermal Reference
  Voltage Sensor : fl_lib/Electrical/Electrical Sensors/Voltage Sensor
  p : PMIOPort  Side=Left
  n : PMIOPort  Port=2  Side=Right
  SOC : Outport
  Current : Outport  Port=2
  Voltage : Outport  Port=3
  Temp : Outport  Port=4
  wires:
  Cell Current (I)/1 -> Current/1, SOC Estimator (Coulomb Counting)/1
  SOC Estimator (Coulomb Counting)/1 -> SOC/1  "Battery State of Charge"
  Constant/1 -> SOC Estimator (Coulomb Counting)/2
  Cell Voltage (V)/1 -> Voltage/1
  Cell Temperature (K)/1 -> Temp/1
  Source Load/1 -> Simulink-PS Converter/1
  connections:
  Temperature Sensor/RConn2 -- Cell Temperature (K)/LConn1
  Voltage Sensor/RConn1 -- Cell Voltage (V)/LConn1
  Temperature Sensor/LConn1 -- Battery Single Particle/RConn2 -- Convective Heat Transfer/LConn1
  Thermal Reference/LConn1 -- Temperature Sensor/RConn1
  Temperature Source/LConn1 -- Convective Heat Transfer/RConn1
  Rs/LConn1 -- Voltage Sensor/LConn1 -- Battery Single Particle/LConn1
  Battery Single Particle/RConn1 -- Voltage Sensor/RConn2 -- Electrical Reference/LConn1 -- Controlled Current Source/LConn1 -- n/RConn1
  Cell Current (I)/LConn1 -- Current Sensor/RConn1
  Current Sensor/LConn1 -- Controlled Current Source/RConn2 -- p/RConn1
  Simulink-PS Converter/RConn1 -- Controlled Current Source/RConn1
  Current Sensor/RConn2 -- Rs/RConn1

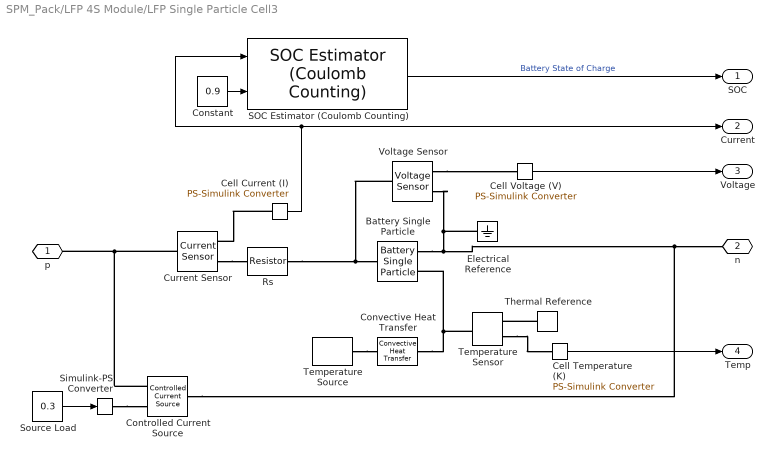
== system SPM_Pack/LFP 4S Module/LFP Single Particle Cell3 ==
  Battery Single Particle : batt_lib/Cells/Electrochemical/Battery Single Particle  ExtrapolationMethod=simscape.enum.extrapolation.nearest  ThicknessAnode=3.4E-5 m  ElectrolyteLayerCountAnode=10  ThicknessSeparator=2.5E-5 m  ElectrolyteLayerCountSeparator=5  ThicknessCathode=8E-5 m  ElectrolyteLayerCountCathode=10  ElectrodePlateArea=0.2 m^2  ParticleRadiusAnode=5E-6 m  ShellCountAnode=30  ParticleRadiusCathode=5E-6 m  ShellCountCathode=30  ActiveMaterialVolumeFractionAnode=0.58  ActiveMaterialVolumeFractionCathode=0.374  OpenCircuitPotentialAnode=[0.200;0.180;0.160;0.140;0.120;0.110;0.102;0.098;0.094;0.092;0.091;0.090;0.089;0.089;0.088;0.088;0.088;0.088;0.088;0.088;0.088;0.087;0.087;0.087;0.086;0.086;0.085;0.085;0.084;0.084;0.083;0.083;0.082;0.082;0.081;0.081;0.080;0.079;0.078] V  OpenCircuitPotentialCathode=[3.200;3.280;3.340;3.380;3.410;3.420;3.425;3.430;3.432;3.433;3.434;3.435;3.435;3.436;3.436;3.437;3.437;3.438;3.438;3.439;3.439;3.440;3.440;3.441;3.441;3.442;3.442;3.443;3.443;3.444;3.444;3.445;3.446;3.447;3.448;3.449;3.460;3.480;3.500] V  NormalizedStoichiometryBreakpoints=linspace(0.025, 0.975, 39)  MaximumConcentrationAnode=30555 mol/m^3  MaximumStoichiometryAnode=0.811  MinimumStoichiometryAnode=0.0132  MaximumConcentrationCathode=22806 mol/m^3  MaximumStoichiometryCathode=0.74  MinimumStoichiometryCathode=0.035  ActiveMaterialDiffusionCoefficientAnode=3E-15 m^2/s  ActiveMaterialDiffusionCoefficientCathode=1E-15 m^2/s  ConductivityAnode=100 S/m  ConductivityCathode=0.5 S/m  CurrentCollectorResistance=1E-3 Ohm  ElectrolyteVolumeFractionAnode=0.3874  ElectrolyteVolumeFractionSeparator=0.45  ElectrolyteVolumeFractionCathode=0.5725  ElectrolyteConductivity=0.29 S/m  BruggemanExponentAnode=1.5  BruggemanExponentSeparator=1.5  BruggemanExponentCathode=1.5  TransferenceNumber=0.363  ElectrolyteDiffusionCoefficient=2E-10 m^2/s  ChargeTransferRateAnode=1E-9 m^(5/2)/(mol^(1/2)*s)  ChargeTransferRateCathode=1E-11 m^(5/2)/(mol^(1/2)*s)  BatteryThermalMass=77 J/K  ArrheniusReferenceTemperature=298.15 K  ActiveMaterialDiffusionActivationEnergyAnode=39000 J/mol  ActiveMaterialDiffusionActivationEnergyCathode=35000 J/mol  ElectrolyteDiffusionActivationEnergy=26600 J/mol  ConductivityActivationEnergyAnode=3000 J/mol  ConductivityActivationEnergyCathode=3000 J/mol  ElectrolyteConductivityActivationEnergy=11000 J/mol  ChargeTransferActivationEnergyAnode=13000 J/mol  ChargeTransferActivationEnergyCathode=20000 J/mol  batteryCurrent_specify=off  batteryCurrent_priority=None  batteryCurrent=0 A  batteryCurrent_nominal_specify=off  batteryCurrent_nominal_value=1  batteryCurrent_nominal_unit=A  batteryVoltage_specify=off  batteryVoltage_priority=None  batteryVoltage=0 V  batteryVoltage_nominal_specify=off  batteryVoltage_nominal_value=1  batteryVoltage_nominal_unit=V  averageElectrolyteConcentration_specify=off  averageElectrolyteConcentration_priority=High  averageElectrolyteConcentration=1200 mol/m^3  averageElectrolyteConcentration_nominal_specify=off  averageElectrolyteConcentration_nominal_value=1  averageElectrolyteConcentration_nominal_unit=mol/m^3  stateOfCharge_specify=off  stateOfCharge_priority=High  stateOfCharge=0.5  stateOfCharge_nominal_specify=off  stateOfCharge_nominal_value=1  stateOfCharge_nominal_unit=1  batteryTemperature_specify=off  batteryTemperature_priority=High  batteryTemperature=298.15 K  batteryTemperature_nominal_specify=off  batteryTemperature_nominal_value=1  batteryTemperature_nominal_unit=K
      settings: InternalSimscapePortConfiguration="{\"Bottom\":[],\"Left\":[{\"id\":\"p\",\"label\":\"+\",\"type\":\"foundation.electrical.electrical\"}],\"Right\":[{\"id\":\"n\",\"label\":\"-\",\"type\":\"foundation.electrical.electrical\"},{\"id\":\"H\",\"label\":\"H\",\"type\":\"foundation.thermal.thermal\"}],\"Top\":[]}"
  Cell Current (I) : nesl_utility/PS-Simulink Converter  PhysicalDomain=network_engine_domain  SubClassName=ps_output  LeftPortType=input  RightPortType=output  PseudoPeriodic=off  Frequencies=[]  VectorFormat=inherit  Unit=A  AffineConversion=off
  Cell Temperature (K) : nesl_utility/PS-Simulink Converter  PhysicalDomain=network_engine_domain  SubClassName=ps_output  LeftPortType=input  RightPortType=output  PseudoPeriodic=off  Frequencies=[]  VectorFormat=inherit  Unit=K  AffineConversion=off
  Cell Voltage (V) : nesl_utility/PS-Simulink Converter  PhysicalDomain=network_engine_domain  SubClassName=ps_output  LeftPortType=input  RightPortType=output  PseudoPeriodic=off  Frequencies=[]  VectorFormat=inherit  Unit=V  AffineConversion=off
  Constant : Constant  Value=0.9
  Controlled Current Source : fl_lib/Electrical/Electrical Sources/Controlled Current Source
  Convective Heat Transfer : fl_lib/Thermal/Thermal Elements/Convective Heat Transfer  thermal_type=foundation.enum.constant_variable.constant  area=0.01 m^2  heat_tr_coeff=15 W/(K*m^2)  min_heat_tr_coeff=1e-3 W/(K*m^2)  T_specify=off  T_priority=None  T=0 K  T_nominal_specify=off  T_nominal_value=1  T_nominal_unit=K  Q_specify=off  Q_priority=None  Q=0 W  Q_nominal_specify=off  Q_nominal_value=1  Q_nominal_unit=W
  Current Sensor : fl_lib/Electrical/Electrical Sensors/Current Sensor
  Electrical Reference : fl_lib/Electrical/Electrical Elements/Electrical Reference
  Rs : fl_lib/Electrical/Electrical Elements/Resistor  R=0.004 Ohm  i_specify=off  i_priority=None  i=0 A  i_nominal_specify=off  i_nominal_value=3  i_nominal_unit=A  v_specify=off  v_priority=None  v=0 V  v_nominal_specify=off  v_nominal_value=3.5  v_nominal_unit=V
  SOC Estimator (Coulomb Counting) : BatteryEstimators/SOC Estimator (Coulomb Counting)  CurrentInputPartition=on  AH=27  Ts=1
      settings: LibrarySourceBlock=|
      | batt_sl_lib/Estimators/SOC Estimator
      | (Coulomb Counting)
  Simulink-PS Converter : nesl_utility/Simulink-PS Converter  PhysicalDomain=network_engine_domain  SubClassName=ps_input  LeftPortType=input  RightPortType=output  PseudoPeriodic=off  Frequencies=[]  NoiseDistribution=none  NoiseParameters=[]  Unit=A  AffineConversion=off  FilteringAndDerivatives=provide  SimscapeFilterOrder=1  InputFilterTimeConstant=0.001  UdotUserProvided=0
  Source Load : Constant  Value=0.3
  Temperature Sensor : fl_lib/Thermal/Thermal Sensors/Temperature Sensor  temperature_measure=foundation.enum.MeasurementReference.difference
  Temperature Source : fl_lib/Thermal/Thermal Sources/Temperature Source  temperature=298.15 K
  Thermal Reference : fl_lib/Thermal/Thermal Elements/Thermal Reference
  Voltage Sensor : fl_lib/Electrical/Electrical Sensors/Voltage Sensor
  p : PMIOPort  Side=Left
  n : PMIOPort  Port=2  Side=Right
  SOC : Outport
  Current : Outport  Port=2
  Voltage : Outport  Port=3
  Temp : Outport  Port=4
  wires:
  Cell Current (I)/1 -> Current/1, SOC Estimator (Coulomb Counting)/1
  SOC Estimator (Coulomb Counting)/1 -> SOC/1  "Battery State of Charge"
  Constant/1 -> SOC Estimator (Coulomb Counting)/2
  Cell Voltage (V)/1 -> Voltage/1
  Cell Temperature (K)/1 -> Temp/1
  Source Load/1 -> Simulink-PS Converter/1
  connections:
  Temperature Sensor/RConn2 -- Cell Temperature (K)/LConn1
  Voltage Sensor/RConn1 -- Cell Voltage (V)/LConn1
  Temperature Sensor/LConn1 -- Battery Single Particle/RConn2 -- Convective Heat Transfer/LConn1
  Thermal Reference/LConn1 -- Temperature Sensor/RConn1
  Temperature Source/LConn1 -- Convective Heat Transfer/RConn1
  Rs/LConn1 -- Voltage Sensor/LConn1 -- Battery Single Particle/LConn1
  Battery Single Particle/RConn1 -- Voltage Sensor/RConn2 -- Electrical Reference/LConn1 -- Controlled Current Source/LConn1 -- n/RConn1
  Cell Current (I)/LConn1 -- Current Sensor/RConn1
  Current Sensor/LConn1 -- Controlled Current Source/RConn2 -- p/RConn1
  Simulink-PS Converter/RConn1 -- Controlled Current Source/RConn1
  Current Sensor/RConn2 -- Rs/RConn1

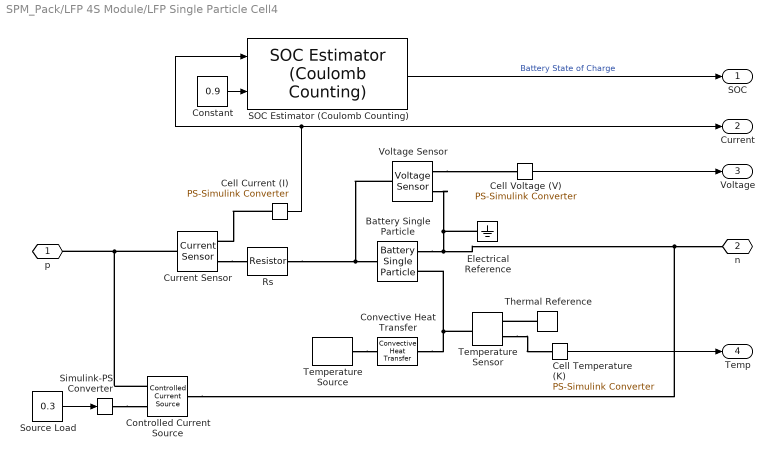
== system SPM_Pack/LFP 4S Module/LFP Single Particle Cell4 ==
  Battery Single Particle : batt_lib/Cells/Electrochemical/Battery Single Particle  ExtrapolationMethod=simscape.enum.extrapolation.nearest  ThicknessAnode=3.4E-5 m  ElectrolyteLayerCountAnode=10  ThicknessSeparator=2.5E-5 m  ElectrolyteLayerCountSeparator=5  ThicknessCathode=8E-5 m  ElectrolyteLayerCountCathode=10  ElectrodePlateArea=0.2 m^2  ParticleRadiusAnode=5E-6 m  ShellCountAnode=30  ParticleRadiusCathode=5E-6 m  ShellCountCathode=30  ActiveMaterialVolumeFractionAnode=0.58  ActiveMaterialVolumeFractionCathode=0.374  OpenCircuitPotentialAnode=[0.200;0.180;0.160;0.140;0.120;0.110;0.102;0.098;0.094;0.092;0.091;0.090;0.089;0.089;0.088;0.088;0.088;0.088;0.088;0.088;0.088;0.087;0.087;0.087;0.086;0.086;0.085;0.085;0.084;0.084;0.083;0.083;0.082;0.082;0.081;0.081;0.080;0.079;0.078] V  OpenCircuitPotentialCathode=[3.200;3.280;3.340;3.380;3.410;3.420;3.425;3.430;3.432;3.433;3.434;3.435;3.435;3.436;3.436;3.437;3.437;3.438;3.438;3.439;3.439;3.440;3.440;3.441;3.441;3.442;3.442;3.443;3.443;3.444;3.444;3.445;3.446;3.447;3.448;3.449;3.460;3.480;3.500] V  NormalizedStoichiometryBreakpoints=linspace(0.025, 0.975, 39)  MaximumConcentrationAnode=30555 mol/m^3  MaximumStoichiometryAnode=0.811  MinimumStoichiometryAnode=0.0132  MaximumConcentrationCathode=22806 mol/m^3  MaximumStoichiometryCathode=0.74  MinimumStoichiometryCathode=0.035  ActiveMaterialDiffusionCoefficientAnode=3E-15 m^2/s  ActiveMaterialDiffusionCoefficientCathode=1E-15 m^2/s  ConductivityAnode=100 S/m  ConductivityCathode=0.5 S/m  CurrentCollectorResistance=1E-3 Ohm  ElectrolyteVolumeFractionAnode=0.3874  ElectrolyteVolumeFractionSeparator=0.45  ElectrolyteVolumeFractionCathode=0.5725  ElectrolyteConductivity=0.29 S/m  BruggemanExponentAnode=1.5  BruggemanExponentSeparator=1.5  BruggemanExponentCathode=1.5  TransferenceNumber=0.363  ElectrolyteDiffusionCoefficient=2E-10 m^2/s  ChargeTransferRateAnode=1E-9 m^(5/2)/(mol^(1/2)*s)  ChargeTransferRateCathode=1E-11 m^(5/2)/(mol^(1/2)*s)  BatteryThermalMass=77 J/K  ArrheniusReferenceTemperature=298.15 K  ActiveMaterialDiffusionActivationEnergyAnode=39000 J/mol  ActiveMaterialDiffusionActivationEnergyCathode=35000 J/mol  ElectrolyteDiffusionActivationEnergy=26600 J/mol  ConductivityActivationEnergyAnode=3000 J/mol  ConductivityActivationEnergyCathode=3000 J/mol  ElectrolyteConductivityActivationEnergy=11000 J/mol  ChargeTransferActivationEnergyAnode=13000 J/mol  ChargeTransferActivationEnergyCathode=20000 J/mol  batteryCurrent_specify=off  batteryCurrent_priority=None  batteryCurrent=0 A  batteryCurrent_nominal_specify=off  batteryCurrent_nominal_value=1  batteryCurrent_nominal_unit=A  batteryVoltage_specify=off  batteryVoltage_priority=None  batteryVoltage=0 V  batteryVoltage_nominal_specify=off  batteryVoltage_nominal_value=1  batteryVoltage_nominal_unit=V  averageElectrolyteConcentration_specify=off  averageElectrolyteConcentration_priority=High  averageElectrolyteConcentration=1200 mol/m^3  averageElectrolyteConcentration_nominal_specify=off  averageElectrolyteConcentration_nominal_value=1  averageElectrolyteConcentration_nominal_unit=mol/m^3  stateOfCharge_specify=off  stateOfCharge_priority=High  stateOfCharge=0.5  stateOfCharge_nominal_specify=off  stateOfCharge_nominal_value=1  stateOfCharge_nominal_unit=1  batteryTemperature_specify=off  batteryTemperature_priority=High  batteryTemperature=298.15 K  batteryTemperature_nominal_specify=off  batteryTemperature_nominal_value=1  batteryTemperature_nominal_unit=K
      settings: InternalSimscapePortConfiguration="{\"Bottom\":[],\"Left\":[{\"id\":\"p\",\"label\":\"+\",\"type\":\"foundation.electrical.electrical\"}],\"Right\":[{\"id\":\"n\",\"label\":\"-\",\"type\":\"foundation.electrical.electrical\"},{\"id\":\"H\",\"label\":\"H\",\"type\":\"foundation.thermal.thermal\"}],\"Top\":[]}"
  Cell Current (I) : nesl_utility/PS-Simulink Converter  PhysicalDomain=network_engine_domain  SubClassName=ps_output  LeftPortType=input  RightPortType=output  PseudoPeriodic=off  Frequencies=[]  VectorFormat=inherit  Unit=A  AffineConversion=off
  Cell Temperature (K) : nesl_utility/PS-Simulink Converter  PhysicalDomain=network_engine_domain  SubClassName=ps_output  LeftPortType=input  RightPortType=output  PseudoPeriodic=off  Frequencies=[]  VectorFormat=inherit  Unit=K  AffineConversion=off
  Cell Voltage (V) : nesl_utility/PS-Simulink Converter  PhysicalDomain=network_engine_domain  SubClassName=ps_output  LeftPortType=input  RightPortType=output  PseudoPeriodic=off  Frequencies=[]  VectorFormat=inherit  Unit=V  AffineConversion=off
  Constant : Constant  Value=0.9
  Controlled Current Source : fl_lib/Electrical/Electrical Sources/Controlled Current Source
  Convective Heat Transfer : fl_lib/Thermal/Thermal Elements/Convective Heat Transfer  thermal_type=foundation.enum.constant_variable.constant  area=0.01 m^2  heat_tr_coeff=15 W/(K*m^2)  min_heat_tr_coeff=1e-3 W/(K*m^2)  T_specify=off  T_priority=None  T=0 K  T_nominal_specify=off  T_nominal_value=1  T_nominal_unit=K  Q_specify=off  Q_priority=None  Q=0 W  Q_nominal_specify=off  Q_nominal_value=1  Q_nominal_unit=W
  Current Sensor : fl_lib/Electrical/Electrical Sensors/Current Sensor
  Electrical Reference : fl_lib/Electrical/Electrical Elements/Electrical Reference
  Rs : fl_lib/Electrical/Electrical Elements/Resistor  R=0.004 Ohm  i_specify=off  i_priority=None  i=0 A  i_nominal_specify=off  i_nominal_value=3  i_nominal_unit=A  v_specify=off  v_priority=None  v=0 V  v_nominal_specify=off  v_nominal_value=3.5  v_nominal_unit=V
  SOC Estimator (Coulomb Counting) : BatteryEstimators/SOC Estimator (Coulomb Counting)  CurrentInputPartition=on  AH=27  Ts=1
      settings: LibrarySourceBlock=|
      | batt_sl_lib/Estimators/SOC Estimator
      | (Coulomb Counting)
  Simulink-PS Converter : nesl_utility/Simulink-PS Converter  PhysicalDomain=network_engine_domain  SubClassName=ps_input  LeftPortType=input  RightPortType=output  PseudoPeriodic=off  Frequencies=[]  NoiseDistribution=none  NoiseParameters=[]  Unit=A  AffineConversion=off  FilteringAndDerivatives=provide  SimscapeFilterOrder=1  InputFilterTimeConstant=0.001  UdotUserProvided=0
  Source Load : Constant  Value=0.3
  Temperature Sensor : fl_lib/Thermal/Thermal Sensors/Temperature Sensor  temperature_measure=foundation.enum.MeasurementReference.difference
  Temperature Source : fl_lib/Thermal/Thermal Sources/Temperature Source  temperature=298.15 K
  Thermal Reference : fl_lib/Thermal/Thermal Elements/Thermal Reference
  Voltage Sensor : fl_lib/Electrical/Electrical Sensors/Voltage Sensor
  p : PMIOPort  Side=Left
  n : PMIOPort  Port=2  Side=Right
  SOC : Outport
  Current : Outport  Port=2
  Voltage : Outport  Port=3
  Temp : Outport  Port=4
  wires:
  Cell Current (I)/1 -> Current/1, SOC Estimator (Coulomb Counting)/1
  SOC Estimator (Coulomb Counting)/1 -> SOC/1  "Battery State of Charge"
  Constant/1 -> SOC Estimator (Coulomb Counting)/2
  Cell Voltage (V)/1 -> Voltage/1
  Cell Temperature (K)/1 -> Temp/1
  Source Load/1 -> Simulink-PS Converter/1
  connections:
  Temperature Sensor/RConn2 -- Cell Temperature (K)/LConn1
  Voltage Sensor/RConn1 -- Cell Voltage (V)/LConn1
  Temperature Sensor/LConn1 -- Battery Single Particle/RConn2 -- Convective Heat Transfer/LConn1
  Thermal Reference/LConn1 -- Temperature Sensor/RConn1
  Temperature Source/LConn1 -- Convective Heat Transfer/RConn1
  Rs/LConn1 -- Voltage Sensor/LConn1 -- Battery Single Particle/LConn1
  Battery Single Particle/RConn1 -- Voltage Sensor/RConn2 -- Electrical Reference/LConn1 -- Controlled Current Source/LConn1 -- n/RConn1
  Cell Current (I)/LConn1 -- Current Sensor/RConn1
  Current Sensor/LConn1 -- Controlled Current Source/RConn2 -- p/RConn1
  Simulink-PS Converter/RConn1 -- Controlled Current Source/RConn1
  Current Sensor/RConn2 -- Rs/RConn1
